simulink model "LGS_allFaultsDeselected"  (R2019b)
settings: Solver=FixedStepDiscrete  StartTime=0.0  StopTime=45.0  FixedStep=0.1  RelTol=1e-3
model workspace (MAT data in the model file):
  fipData : object (value not decoded)
  fipName : object (value not decoded)
  stepSize = 0.1
libraries: LibFaultInjectionControls x190, commrandsrc3 x70, simulink x3, LibFailureCondition x1
(part 4 of 41)

== system LGS_allFaultsDeselected/sensor up down handle/FIP2 ==
  In1 : Inport
  Handle sensor FIP2 : Subsystem  mask(FailureInjectionPoint){}
      mask help: FailureInjectionPoint
      mask init: same as LGS_allFaultsDeselected/Analogical switch and general electro-valve and pressure sensor/Analogical switch/Analog Switch FIP
      settings: OpenFcn=|
      | open_system(gcb,'mask');
      | 
      | treeValues = FailureInjectionPointHelper.getAllFmAndParamsAsTreeString(gcb);
      | mo = Simulink.Mask.get(gcb);
      | dc = mo.getDialogControl('GbFmInfo');
      | treeView = dc.getDialogControl('TreeViewFM');
      | treeView.TreeItems = {};
      | treeView.TreeItems = treeValues;
      mask Help: FailureInjectionPoint
      mask DialogControl Control7 Prompt: Containing Failure Modes
      mask DialogControl BtnMoveUp Prompt: Move up
      mask DialogControl BtnMoveUp Callback:
      | %Get name of the failure mode block
      | mo = Simulink.Mask.get(gcb);
      | dc = mo.getDialogControl('GbFmInfo');
      | treeView = dc.getDialogControl('TreeViewFM');
      | try
      |     a = treeView.getSelectedItems();
      |     p = split(a, '/'); %name of failure mode block is p{1}
      | catch
      |     return;
      | end
      | 
      | %Save port handles
      | lh = get_param([gcb,'/',p{1}],'LineHandles');
      | ph = get_param([gcb,'/',p{1}],'PortHandles');
      | this_in = ph.Inport(1);
      | this_out = ph.Outport(1);
      | 
      | last_block = get_param(lh.Inport(1),'SrcBlockHandle');
      | last_block_type = get_param(last_block,'BlockType');
      | if strcmp(last_block_type,'Inport')
      |     return;
      | end
      | lb_lh = get_param(last_block,'LineHandles');
      | 
      | last_out = get_param(lh.Inport(1),'SrcPortHandle');
      | last_in = get_param(lb_lh.Inport(1),'DstPortHandle');
      | next_to_last_out = get_param(lb_lh.Inport(1),'SrcPortHandle');
      | next_in = get_param(lh.Outport(1),'DstPortHandle');
      | 
      | %Delete connecting lines
      | delete_line(lh.Inport(1));
      | delete_line(lh.Outport(1));
      | delete_line(lb_lh.Inport(1));
      | 
      | % Generate new lines
      | add_line(gcb, last_out, next_in, 'autorouting', 'smart');
      | add_line(gcb, this_out, last_in, 'autorouting', 'smart');
      | add_line(gcb, next_to_last_out, this_in, 'autorouting', 'smart');
      | 
      | %Rearrange system
      | Simulink.BlockDiagram.arrangeSystem(gcb);
      | 
      | %Refresh
      | treeValues = FailureInjectionPointHelper.getAllFmAndParamsAsTreeString(gcb);
      | mo = Simulink.Mask.get(gcb);
      | dc = mo.getDialogControl('GbFmInfo');
      | treeView = dc.getDialogControl('TreeViewFM');
      | treeView.TreeItems = {};
      | treeView.TreeItems = treeValues;
      mask DialogControl BtnMoveDown Prompt: Move down
      mask DialogControl BtnMoveDown Callback:
      | %Get name of the failure mode block
      | mo = Simulink.Mask.get(gcb);
      | dc = mo.getDialogControl('GbFmInfo');
      | treeView = dc.getDialogControl('TreeViewFM');
      | try
      |     a = treeView.getSelectedItems();
      |     p = split(a, '/'); %name of failure mode block is p{1}
      | catch
      |     return;
      | end
      | 
      | %Save port handles
      | lh = get_param([gcb,'/',p{1}],'LineHandles');
      | ph = get_param([gcb,'/',p{1}],'PortHandles');
      | this_in = ph.Inport(1);
      | this_out = ph.Outport(1);
      | 
      | next_block = get_param(lh.Outport(1),'DstBlockHandle');
      | next_block_type = get_param(next_block,'BlockType');
      | if strcmp(next_block_type,'Outport')
      |     return;
      | end
      | nb_lh = get_param(next_block,'LineHandles');
      | 
      | last_out = get_param(lh.Inport(1),'SrcPortHandle');
      | next_out = get_param(nb_lh.Outport(1),'SrcPortHandle');
      | next_but_one_in = get_param(nb_lh.Outport(1),'DstPortHandle');
      | next_in = get_param(lh.Outport(1),'DstPortHandle');
      | 
      | %Delete connecting lines
      | delete_line(lh.Inport(1));
      | delete_line(lh.Outport(1));
      | delete_line(nb_lh.Outport(1));
      | 
      | % Generate new lines
      | add_line(gcb, last_out, next_in, 'autorouting', 'smart');
      | add_line(gcb, next_out, this_in, 'autorouting', 'smart');
      | add_line(gcb, this_out, next_but_one_in, 'autorouting', 'smart');
      | 
      | %Rearrange system
      | Simulink.BlockDiagram.arrangeSystem(gcb);
      | 
      | %Refresh
      | treeValues = FailureInjectionPointHelper.getAllFmAndParamsAsTreeString(gcb);
      | mo = Simulink.Mask.get(gcb);
      | dc = mo.getDialogControl('GbFmInfo');
      | treeView = dc.getDialogControl('TreeViewFM');
      | treeView.TreeItems = {};
      | treeView.TreeItems = treeValues;
      mask DialogControl TreeViewFM Prompt: Failure Mode Information
      mask DialogControl BtnOpen Prompt: Open FIP
      mask DialogControl BtnOpen Callback: open_system(gcb,'force');
      mask DialogControl BtnNew Prompt: New
      mask DialogControl BtnNew Callback:
      | dialog_fipManager_single(gcb, '');
      | 
      | %Enable move, edit, delete buttons
      | mo = Simulink.Mask.get(gcb);
      | mo.getDialogControl('BtnMoveUp').Enabled = 'on';
      | mo.getDialogControl('BtnMoveDown').Enabled = 'on';
      | mo.getDialogControl('BtnEdit').Enabled = 'on';
      | mo.getDialogControl('BtnDelete').Enabled = 'on';
      mask DialogControl BtnEdit Prompt: Edit
      mask DialogControl BtnEdit Callback:
      | mo = Simulink.Mask.get(gcb);
      | dc = mo.getDialogControl('GbFmInfo');
      | treeView = dc.getDialogControl('TreeViewFM');
      | try
      |     a = treeView.getSelectedItems();
      |     p = split(a, '/');
      | catch
      |     return;
      | end
      | dialog_fipManager_single(gcb, p{1});
      mask DialogControl BtnDelete Prompt: Delete
      mask DialogControl BtnDelete Callback:
      | %Get name of the failure mode block
      | mo = Simulink.Mask.get(gcb);
      | dc = mo.getDialogControl('GbFmInfo');
      | treeView = dc.getDialogControl('TreeViewFM');
      | try
      |     a = treeView.getSelectedItems();
      |     p = split(a, '/'); %name of failure mode block is p{1}
      | catch
      |     return;
      | end
      | 
      | %Save outport handle of the last and inport handle of the next block
      | lh = get_param([gcb,'/',p{1}],'LineHandles');
      | last_out = get_param(lh.Inport(1),'SrcPortHandle');
      | next_in = get_param(lh.Outport(1),'DstPortHandle');
      | 
      | %Delete connecting lines and failure mode block
      | delete_line(lh.Inport(1));
      | delete_line(lh.Outport(1));
      | fm_handle = get_param([gcb,'/',p{1}],'Handle');
      | delete_block(fm_handle);
      | 
      | % Generate new line from outport last to inport next
      | add_line(gcb, last_out, next_in, 'autorouting', 'smart');
      | 
      | %Rearrange system
      | Simulink.BlockDiagram.arrangeSystem(gcb);
      | 
      | %Disable move, edit, delete buttons in case all FMs are deleted
      | last_block = get_param(last_out,'Parent');
      | last_is_inport = strcmp(get_param(last_block,'BlockType'),'Inport');
      | next_block = get_param(next_in,'Parent');
      | next_is_outport = strcmp(get_param(next_block,'BlockType'),'Outport');
      | if (last_is_inport && next_is_outport)
      |     mo.getDialogControl('BtnMoveUp').Enabled = 'off';
      |     mo.getDialogControl('BtnMoveDown').Enabled = 'off';
      |     mo.getDialogControl('BtnEdit').Enabled = 'off';
      |     mo.getDialogControl('BtnDelete').Enabled = 'off';
      | end
      | 
      | %Refresh
      | treeValues = FailureInjectionPointHelper.getAllFmAndParamsAsTreeString(gcb);
      | mo = Simulink.Mask.get(gcb);
      | dc = mo.getDialogControl('GbFmInfo');
      | treeView = dc.getDialogControl('TreeViewFM');
      | treeView.TreeItems = {};
      | treeView.TreeItems = treeValues;
      mask DialogControl BtnRefresh Prompt: Refresh
      mask DialogControl BtnRefresh Callback:
      | set_param(gcb,'LinkStatus','none');
      | 
      | treeValues = FailureInjectionPointHelper.getAllFmAndParamsAsTreeString(gcb);
      | mo = Simulink.Mask.get(gcb);
      | dc = mo.getDialogControl('GbFmInfo');
      | treeView = dc.getDialogControl('TreeViewFM');
      | treeView.TreeItems = {};
      | treeView.TreeItems = treeValues;
      mask Display: image('icons/failure_injection_point.png','center')
  Out1 : Outport
  wires:
  In1/1 -> Handle sensor FIP2/1(In1)
  Handle sensor FIP2/1(Out1) -> Out1/1

== system LGS_allFaultsDeselected/sensor up down handle/FIP3 ==
  In1 : Inport
  Handle sensor FIP3 : Subsystem  mask(FailureInjectionPoint){}
      mask help: FailureInjectionPoint
      mask init: same as LGS_allFaultsDeselected/Analogical switch and general electro-valve and pressure sensor/Analogical switch/Analog Switch FIP
      settings: OpenFcn=|
      | open_system(gcb,'mask');
      | 
      | treeValues = FailureInjectionPointHelper.getAllFmAndParamsAsTreeString(gcb);
      | mo = Simulink.Mask.get(gcb);
      | dc = mo.getDialogControl('GbFmInfo');
      | treeView = dc.getDialogControl('TreeViewFM');
      | treeView.TreeItems = {};
      | treeView.TreeItems = treeValues;
      mask Help: FailureInjectionPoint
      mask DialogControl Control7 Prompt: Containing Failure Modes
      mask DialogControl BtnMoveUp Prompt: Move up
      mask DialogControl BtnMoveUp Callback:
      | %Get name of the failure mode block
      | mo = Simulink.Mask.get(gcb);
      | dc = mo.getDialogControl('GbFmInfo');
      | treeView = dc.getDialogControl('TreeViewFM');
      | try
      |     a = treeView.getSelectedItems();
      |     p = split(a, '/'); %name of failure mode block is p{1}
      | catch
      |     return;
      | end
      | 
      | %Save port handles
      | lh = get_param([gcb,'/',p{1}],'LineHandles');
      | ph = get_param([gcb,'/',p{1}],'PortHandles');
      | this_in = ph.Inport(1);
      | this_out = ph.Outport(1);
      | 
      | last_block = get_param(lh.Inport(1),'SrcBlockHandle');
      | last_block_type = get_param(last_block,'BlockType');
      | if strcmp(last_block_type,'Inport')
      |     return;
      | end
      | lb_lh = get_param(last_block,'LineHandles');
      | 
      | last_out = get_param(lh.Inport(1),'SrcPortHandle');
      | last_in = get_param(lb_lh.Inport(1),'DstPortHandle');
      | next_to_last_out = get_param(lb_lh.Inport(1),'SrcPortHandle');
      | next_in = get_param(lh.Outport(1),'DstPortHandle');
      | 
      | %Delete connecting lines
      | delete_line(lh.Inport(1));
      | delete_line(lh.Outport(1));
      | delete_line(lb_lh.Inport(1));
      | 
      | % Generate new lines
      | add_line(gcb, last_out, next_in, 'autorouting', 'smart');
      | add_line(gcb, this_out, last_in, 'autorouting', 'smart');
      | add_line(gcb, next_to_last_out, this_in, 'autorouting', 'smart');
      | 
      | %Rearrange system
      | Simulink.BlockDiagram.arrangeSystem(gcb);
      | 
      | %Refresh
      | treeValues = FailureInjectionPointHelper.getAllFmAndParamsAsTreeString(gcb);
      | mo = Simulink.Mask.get(gcb);
      | dc = mo.getDialogControl('GbFmInfo');
      | treeView = dc.getDialogControl('TreeViewFM');
      | treeView.TreeItems = {};
      | treeView.TreeItems = treeValues;
      mask DialogControl BtnMoveDown Prompt: Move down
      mask DialogControl BtnMoveDown Callback:
      | %Get name of the failure mode block
      | mo = Simulink.Mask.get(gcb);
      | dc = mo.getDialogControl('GbFmInfo');
      | treeView = dc.getDialogControl('TreeViewFM');
      | try
      |     a = treeView.getSelectedItems();
      |     p = split(a, '/'); %name of failure mode block is p{1}
      | catch
      |     return;
      | end
      | 
      | %Save port handles
      | lh = get_param([gcb,'/',p{1}],'LineHandles');
      | ph = get_param([gcb,'/',p{1}],'PortHandles');
      | this_in = ph.Inport(1);
      | this_out = ph.Outport(1);
      | 
      | next_block = get_param(lh.Outport(1),'DstBlockHandle');
      | next_block_type = get_param(next_block,'BlockType');
      | if strcmp(next_block_type,'Outport')
      |     return;
      | end
      | nb_lh = get_param(next_block,'LineHandles');
      | 
      | last_out = get_param(lh.Inport(1),'SrcPortHandle');
      | next_out = get_param(nb_lh.Outport(1),'SrcPortHandle');
      | next_but_one_in = get_param(nb_lh.Outport(1),'DstPortHandle');
      | next_in = get_param(lh.Outport(1),'DstPortHandle');
      | 
      | %Delete connecting lines
      | delete_line(lh.Inport(1));
      | delete_line(lh.Outport(1));
      | delete_line(nb_lh.Outport(1));
      | 
      | % Generate new lines
      | add_line(gcb, last_out, next_in, 'autorouting', 'smart');
      | add_line(gcb, next_out, this_in, 'autorouting', 'smart');
      | add_line(gcb, this_out, next_but_one_in, 'autorouting', 'smart');
      | 
      | %Rearrange system
      | Simulink.BlockDiagram.arrangeSystem(gcb);
      | 
      | %Refresh
      | treeValues = FailureInjectionPointHelper.getAllFmAndParamsAsTreeString(gcb);
      | mo = Simulink.Mask.get(gcb);
      | dc = mo.getDialogControl('GbFmInfo');
      | treeView = dc.getDialogControl('TreeViewFM');
      | treeView.TreeItems = {};
      | treeView.TreeItems = treeValues;
      mask DialogControl TreeViewFM Prompt: Failure Mode Information
      mask DialogControl BtnOpen Prompt: Open FIP
      mask DialogControl BtnOpen Callback: open_system(gcb,'force');
      mask DialogControl BtnNew Prompt: New
      mask DialogControl BtnNew Callback:
      | dialog_fipManager_single(gcb, '');
      | 
      | %Enable move, edit, delete buttons
      | mo = Simulink.Mask.get(gcb);
      | mo.getDialogControl('BtnMoveUp').Enabled = 'on';
      | mo.getDialogControl('BtnMoveDown').Enabled = 'on';
      | mo.getDialogControl('BtnEdit').Enabled = 'on';
      | mo.getDialogControl('BtnDelete').Enabled = 'on';
      mask DialogControl BtnEdit Prompt: Edit
      mask DialogControl BtnEdit Callback:
      | mo = Simulink.Mask.get(gcb);
      | dc = mo.getDialogControl('GbFmInfo');
      | treeView = dc.getDialogControl('TreeViewFM');
      | try
      |     a = treeView.getSelectedItems();
      |     p = split(a, '/');
      | catch
      |     return;
      | end
      | dialog_fipManager_single(gcb, p{1});
      mask DialogControl BtnDelete Prompt: Delete
      mask DialogControl BtnDelete Callback:
      | %Get name of the failure mode block
      | mo = Simulink.Mask.get(gcb);
      | dc = mo.getDialogControl('GbFmInfo');
      | treeView = dc.getDialogControl('TreeViewFM');
      | try
      |     a = treeView.getSelectedItems();
      |     p = split(a, '/'); %name of failure mode block is p{1}
      | catch
      |     return;
      | end
      | 
      | %Save outport handle of the last and inport handle of the next block
      | lh = get_param([gcb,'/',p{1}],'LineHandles');
      | last_out = get_param(lh.Inport(1),'SrcPortHandle');
      | next_in = get_param(lh.Outport(1),'DstPortHandle');
      | 
      | %Delete connecting lines and failure mode block
      | delete_line(lh.Inport(1));
      | delete_line(lh.Outport(1));
      | fm_handle = get_param([gcb,'/',p{1}],'Handle');
      | delete_block(fm_handle);
      | 
      | % Generate new line from outport last to inport next
      | add_line(gcb, last_out, next_in, 'autorouting', 'smart');
      | 
      | %Rearrange system
      | Simulink.BlockDiagram.arrangeSystem(gcb);
      | 
      | %Disable move, edit, delete buttons in case all FMs are deleted
      | last_block = get_param(last_out,'Parent');
      | last_is_inport = strcmp(get_param(last_block,'BlockType'),'Inport');
      | next_block = get_param(next_in,'Parent');
      | next_is_outport = strcmp(get_param(next_block,'BlockType'),'Outport');
      | if (last_is_inport && next_is_outport)
      |     mo.getDialogControl('BtnMoveUp').Enabled = 'off';
      |     mo.getDialogControl('BtnMoveDown').Enabled = 'off';
      |     mo.getDialogControl('BtnEdit').Enabled = 'off';
      |     mo.getDialogControl('BtnDelete').Enabled = 'off';
      | end
      | 
      | %Refresh
      | treeValues = FailureInjectionPointHelper.getAllFmAndParamsAsTreeString(gcb);
      | mo = Simulink.Mask.get(gcb);
      | dc = mo.getDialogControl('GbFmInfo');
      | treeView = dc.getDialogControl('TreeViewFM');
      | treeView.TreeItems = {};
      | treeView.TreeItems = treeValues;
      mask DialogControl BtnRefresh Prompt: Refresh
      mask DialogControl BtnRefresh Callback:
      | set_param(gcb,'LinkStatus','none');
      | 
      | treeValues = FailureInjectionPointHelper.getAllFmAndParamsAsTreeString(gcb);
      | mo = Simulink.Mask.get(gcb);
      | dc = mo.getDialogControl('GbFmInfo');
      | treeView = dc.getDialogControl('TreeViewFM');
      | treeView.TreeItems = {};
      | treeView.TreeItems = treeValues;
      mask Display: image('icons/failure_injection_point.png','center')
  Out1 : Outport
  wires:
  In1/1 -> Handle sensor FIP3/1(In1)
  Handle sensor FIP3/1(Out1) -> Out1/1

== system LGS_allFaultsDeselected/Analogical switch and general electro-valve and pressure sensor/Analogical switch/Analog Switch FIP ==
  In1 : Inport
  Blocked closed : Subsystem  mask(FailureMode){isActive=off, isDSF=off, Value=true, FailureRate=1.0E-3, useDefaultMt_copy=off, MaintenanceTask=0, useDefaultMt=off, RiskTime=0, useDefaultRt=off, File=[], DSFjson=JSON}
      mask prompts: isActive "is Active"; isDSF "DSF Trigger"; Value "Bool Value"; useDefaultMt_copy "set"; useDefaultMt "set"; useDefaultRt "set"
      mask TypeOptions isActive: Trigger FIP/Active
      mask TypeOptions isDSF: Trigger FIP/isDSF
      mask Callback isDSF:
      | a = Simulink.Mask.get(gcb);
      | disp(a);
      | d = a.DialogControls();
      | disp(d);
      | for i = 1:size(d,2)
      |     if strcmp(d(i).Name, 'ParameterGroupVar')
      |         basicFip_ctrl = d(i).getDialogControl('BasicFipParam');
      |         dsFip_ctrl = d(i).getDialogControl('DSFipParam');
      | 
      |         if strcmp(get_param(gcb, 'isDSF'), 'on')
      | %            basicFip_ctrl.Visible = 'off';
      |             basicFip_ctrl.Enabled = 'off';
      | 
      |             dsFip_ctrl.Enabled = 'on';
      | %            dsFip_ctrl.Visible = 'on';
      |         else
      |             basicFip_ctrl.Enabled = 'on';
      | %            basicFip_ctrl.Visible = 'on';
      | 
      | %            dsFip_ctrl.Visible = 'off';
      |             dsFip_ctrl.Enabled = 'off';
      |         end
      |     end
      | end
      mask TypeOptions Value: CommitValue/Value
      mask TypeOptions FailureRate: Trigger FIP/FailureRate
      mask Callback useDefaultMt_copy:
      | a = Simulink.Mask.get(gcb);
      | d = a.Parameters();
      | for i = 1:size(d,2)
      |     if strcmp(d(i).Name, 'MaintenanceTask')
      |         if strcmp(get_param(gcb, 'useDefaultMt'), 'off')
      |             set_param(gcb,'MaintenanceTask', '0')
      |             d(i).Enabled = 'off';
      |         else
      |             d(i).Enabled = 'on';
      |         end
      |     end
      | end
      mask TypeOptions MaintenanceTask: Trigger FIP/MaintenanceTask
      mask Callback useDefaultMt:
      | a = Simulink.Mask.get(gcb);
      | d = a.Parameters();
      | for i = 1:size(d,2)
      |     if strcmp(d(i).Name, 'MaintenanceTask')
      |         if strcmp(get_param(gcb, 'useDefaultMt'), 'off')
      |             set_param(gcb,'MaintenanceTask', '0')
      |             d(i).Enabled = 'off';
      |         else
      |             d(i).Enabled = 'on';
      |         end
      |     end
      | end
      mask TypeOptions RiskTime: Trigger FIP/RiskTime
      mask Callback useDefaultRt:
      | a = Simulink.Mask.get(gcb);
      | d = a.Parameters();
      | for i = 1:size(d,2)
      |     if strcmp(d(i).Name, 'RiskTime')
      |         if strcmp(get_param(gcb, 'useDefaultRt'), 'off')
      |             set_param(gcb,'RiskTime', '0')
      |             d(i).Enabled = 'off';
      |         else
      |             d(i).Enabled = 'on';
      |         end
      |     end
      | end
      mask TypeOptions DSFjson: Trigger FIP/DSFjson
      mask DialogControl DescGroupVar Prompt: Bool
      mask DialogControl DescTextVar Prompt: Controls for a fault with boolean as result type
      mask DialogControl BasicFipBehavior Prompt: Failure Mode Behavior
      mask DialogControl BasicFipParamTab Prompt: Failure Mode Occurrence
      mask DialogControl BasicFipParam Prompt: Parameters
      mask DialogControl FailureRate_label Prompt: Failure Rate [1/h]
      mask DialogControl MaintenanceTask_label Prompt: Maintenance Task [h]
      mask DialogControl RiskTime_label Prompt: Risk time [h]
      mask DialogControl DSFipParamTab Prompt: Dependent System Information
      mask DialogControl DSFipParam Prompt: Parameters
      mask DialogControl LoadCSV Prompt: Browse
      mask DialogControl LoadCSV Callback:
      | [file,path,indx] = uigetfile('*.csv');
      | try
      |     set_param(gcb, 'File', append(path,file));
      |     file = fopen(append(path,file));
      | 
      |     fips = {};
      |     cutsets = {};
      | 
      |     line = fgetl(file);
      |     while ischar(line)
      |         disp(join([' > Processing: ',line]));
      |         splitString = split(line, ';');
      |         if isequal(splitString{1}, 'Cut set')
      |             disp('   > Found Cut set');
      |             cs = splitString(2:end-1);
      |             disp(cs);
      |             cutsets{end+1} = cs';
      |         else
      |             disp('   > Found FIP');
      |             if ~isequal("h", splitString(7))
      |                 disp('no time format except hour is supported');
      |             end
      |             fip = {};
      |             fip.id = splitString(1);
      |             fip.path = splitString(3);
      |             fip.rate = splitString(4);
      |             fip.checkInterval = splitString(6);
      |             disp(fip);
      |             fips{end+1} = fip;
      |         end
      |         line = fgetl(file);
      |     end
      | 
      |     fclose(file);
      | 
      |     DSF = {};
      |     DSF.fips = fips;
      |     DSF.cutsets = cutsets;
      | 
      |     VarCSText = jsonencode(DSF);
      |     set_param(gcb, 'DSFjson', VarCSText);
      | catch
      | end
  Blocked open : Subsystem  mask(FailureMode){isActive=off, isDSF=off, Value=false, FailureRate=1.0E-3, useDefaultMt_copy=off, MaintenanceTask=0, useDefaultMt=off, RiskTime=0, useDefaultRt=off, File=[], DSFjson=JSON}
      mask prompts: isActive "is Active"; isDSF "DSF Trigger"; Value "Bool Value"; useDefaultMt_copy "set"; useDefaultMt "set"; useDefaultRt "set"
      mask TypeOptions isActive: Trigger FIP/Active
      mask TypeOptions isDSF: Trigger FIP/isDSF
      mask Callback isDSF:
      | a = Simulink.Mask.get(gcb);
      | disp(a);
      | d = a.DialogControls();
      | disp(d);
      | for i = 1:size(d,2)
      |     if strcmp(d(i).Name, 'ParameterGroupVar')
      |         basicFip_ctrl = d(i).getDialogControl('BasicFipParam');
      |         dsFip_ctrl = d(i).getDialogControl('DSFipParam');
      | 
      |         if strcmp(get_param(gcb, 'isDSF'), 'on')
      | %            basicFip_ctrl.Visible = 'off';
      |             basicFip_ctrl.Enabled = 'off';
      | 
      |             dsFip_ctrl.Enabled = 'on';
      | %            dsFip_ctrl.Visible = 'on';
      |         else
      |             basicFip_ctrl.Enabled = 'on';
      | %            basicFip_ctrl.Visible = 'on';
      | 
      | %            dsFip_ctrl.Visible = 'off';
      |             dsFip_ctrl.Enabled = 'off';
      |         end
      |     end
      | end
      mask TypeOptions Value: CommitValue/Value
      mask TypeOptions FailureRate: Trigger FIP/FailureRate
      mask Callback useDefaultMt_copy:
      | a = Simulink.Mask.get(gcb);
      | d = a.Parameters();
      | for i = 1:size(d,2)
      |     if strcmp(d(i).Name, 'MaintenanceTask')
      |         if strcmp(get_param(gcb, 'useDefaultMt'), 'off')
      |             set_param(gcb,'MaintenanceTask', '0')
      |             d(i).Enabled = 'off';
      |         else
      |             d(i).Enabled = 'on';
      |         end
      |     end
      | end
      mask TypeOptions MaintenanceTask: Trigger FIP/MaintenanceTask
      mask Callback useDefaultMt:
      | a = Simulink.Mask.get(gcb);
      | d = a.Parameters();
      | for i = 1:size(d,2)
      |     if strcmp(d(i).Name, 'MaintenanceTask')
      |         if strcmp(get_param(gcb, 'useDefaultMt'), 'off')
      |             set_param(gcb,'MaintenanceTask', '0')
      |             d(i).Enabled = 'off';
      |         else
      |             d(i).Enabled = 'on';
      |         end
      |     end
      | end
      mask TypeOptions RiskTime: Trigger FIP/RiskTime
      mask Callback useDefaultRt:
      | a = Simulink.Mask.get(gcb);
      | d = a.Parameters();
      | for i = 1:size(d,2)
      |     if strcmp(d(i).Name, 'RiskTime')
      |         if strcmp(get_param(gcb, 'useDefaultRt'), 'off')
      |             set_param(gcb,'RiskTime', '0')
      |             d(i).Enabled = 'off';
      |         else
      |             d(i).Enabled = 'on';
      |         end
      |     end
      | end
      mask TypeOptions DSFjson: Trigger FIP/DSFjson
      mask DialogControl DescGroupVar Prompt: Bool
      mask DialogControl DescTextVar Prompt: Controls for a fault with boolean as result type
      mask DialogControl BasicFipBehavior Prompt: Failure Mode Behavior
      mask DialogControl BasicFipParamTab Prompt: Failure Mode Occurrence
      mask DialogControl BasicFipParam Prompt: Parameters
      mask DialogControl FailureRate_label Prompt: Failure Rate [1/h]
      mask DialogControl MaintenanceTask_label Prompt: Maintenance Task [h]
      mask DialogControl RiskTime_label Prompt: Risk time [h]
      mask DialogControl DSFipParamTab Prompt: Dependent System Information
      mask DialogControl DSFipParam Prompt: Parameters
      mask DialogControl LoadCSV Prompt: Browse
      mask DialogControl LoadCSV Callback:
      | [file,path,indx] = uigetfile('*.csv');
      | try
      |     set_param(gcb, 'File', append(path,file));
      |     file = fopen(append(path,file));
      | 
      |     fips = {};
      |     cutsets = {};
      | 
      |     line = fgetl(file);
      |     while ischar(line)
      |         disp(join([' > Processing: ',line]));
      |         splitString = split(line, ';');
      |         if isequal(splitString{1}, 'Cut set')
      |             disp('   > Found Cut set');
      |             cs = splitString(2:end-1);
      |             disp(cs);
      |             cutsets{end+1} = cs';
      |         else
      |             disp('   > Found FIP');
      |             if ~isequal("h", splitString(7))
      |                 disp('no time format except hour is supported');
      |             end
      |             fip = {};
      |             fip.id = splitString(1);
      |             fip.path = splitString(3);
      |             fip.rate = splitString(4);
      |             fip.checkInterval = splitString(6);
      |             disp(fip);
      |             fips{end+1} = fip;
      |         end
      |         line = fgetl(file);
      |     end
      | 
      |     fclose(file);
      | 
      |     DSF = {};
      |     DSF.fips = fips;
      |     DSF.cutsets = cutsets;
      | 
      |     VarCSText = jsonencode(DSF);
      |     set_param(gcb, 'DSFjson', VarCSText);
      | catch
      | end
  Out1 : Outport
  wires:
  Blocked closed/1(Out1) -> Blocked open/1(In1)
  In1/1 -> Blocked closed/1(In1)
  Blocked open/1(Out1) -> Out1/1

== system LGS_allFaultsDeselected/Analogical switch and general electro-valve and pressure sensor/General EV/General EV FIP ==
  In1 : Inport
  Blocked closed : Subsystem  mask(FailureMode){isActive=off, isDSF=off, Value=false, FailureRate=1.0E-3, useDefaultMt_copy=off, MaintenanceTask=0, useDefaultMt=off, RiskTime=0, useDefaultRt=off, File=[], DSFjson=JSON}
      mask prompts: isActive "is Active"; isDSF "DSF Trigger"; Value "Bool Value"; useDefaultMt_copy "set"; useDefaultMt "set"; useDefaultRt "set"
      mask TypeOptions isActive: Trigger FIP/Active
      mask TypeOptions isDSF: Trigger FIP/isDSF
      mask Callback isDSF:
      | a = Simulink.Mask.get(gcb);
      | disp(a);
      | d = a.DialogControls();
      | disp(d);
      | for i = 1:size(d,2)
      |     if strcmp(d(i).Name, 'ParameterGroupVar')
      |         basicFip_ctrl = d(i).getDialogControl('BasicFipParam');
      |         dsFip_ctrl = d(i).getDialogControl('DSFipParam');
      | 
      |         if strcmp(get_param(gcb, 'isDSF'), 'on')
      | %            basicFip_ctrl.Visible = 'off';
      |             basicFip_ctrl.Enabled = 'off';
      | 
      |             dsFip_ctrl.Enabled = 'on';
      | %            dsFip_ctrl.Visible = 'on';
      |         else
      |             basicFip_ctrl.Enabled = 'on';
      | %            basicFip_ctrl.Visible = 'on';
      | 
      | %            dsFip_ctrl.Visible = 'off';
      |             dsFip_ctrl.Enabled = 'off';
      |         end
      |     end
      | end
      mask TypeOptions Value: CommitValue/Value
      mask TypeOptions FailureRate: Trigger FIP/FailureRate
      mask Callback useDefaultMt_copy:
      | a = Simulink.Mask.get(gcb);
      | d = a.Parameters();
      | for i = 1:size(d,2)
      |     if strcmp(d(i).Name, 'MaintenanceTask')
      |         if strcmp(get_param(gcb, 'useDefaultMt'), 'off')
      |             set_param(gcb,'MaintenanceTask', '0')
      |             d(i).Enabled = 'off';
      |         else
      |             d(i).Enabled = 'on';
      |         end
      |     end
      | end
      mask TypeOptions MaintenanceTask: Trigger FIP/MaintenanceTask
      mask Callback useDefaultMt:
      | a = Simulink.Mask.get(gcb);
      | d = a.Parameters();
      | for i = 1:size(d,2)
      |     if strcmp(d(i).Name, 'MaintenanceTask')
      |         if strcmp(get_param(gcb, 'useDefaultMt'), 'off')
      |             set_param(gcb,'MaintenanceTask', '0')
      |             d(i).Enabled = 'off';
      |         else
      |             d(i).Enabled = 'on';
      |         end
      |     end
      | end
      mask TypeOptions RiskTime: Trigger FIP/RiskTime
      mask Callback useDefaultRt:
      | a = Simulink.Mask.get(gcb);
      | d = a.Parameters();
      | for i = 1:size(d,2)
      |     if strcmp(d(i).Name, 'RiskTime')
      |         if strcmp(get_param(gcb, 'useDefaultRt'), 'off')
      |             set_param(gcb,'RiskTime', '0')
      |             d(i).Enabled = 'off';
      |         else
      |             d(i).Enabled = 'on';
      |         end
      |     end
      | end
      mask TypeOptions DSFjson: Trigger FIP/DSFjson
      mask DialogControl DescGroupVar Prompt: Bool
      mask DialogControl DescTextVar Prompt: Controls for a fault with boolean as result type
      mask DialogControl BasicFipBehavior Prompt: Failure Mode Behavior
      mask DialogControl BasicFipParamTab Prompt: Failure Mode Occurrence
      mask DialogControl BasicFipParam Prompt: Parameters
      mask DialogControl FailureRate_label Prompt: Failure Rate [1/h]
      mask DialogControl MaintenanceTask_label Prompt: Maintenance Task [h]
      mask DialogControl RiskTime_label Prompt: Risk time [h]
      mask DialogControl DSFipParamTab Prompt: Dependent System Information
      mask DialogControl DSFipParam Prompt: Parameters
      mask DialogControl LoadCSV Prompt: Browse
      mask DialogControl LoadCSV Callback:
      | [file,path,indx] = uigetfile('*.csv');
      | try
      |     set_param(gcb, 'File', append(path,file));
      |     file = fopen(append(path,file));
      | 
      |     fips = {};
      |     cutsets = {};
      | 
      |     line = fgetl(file);
      |     while ischar(line)
      |         disp(join([' > Processing: ',line]));
      |         splitString = split(line, ';');
      |         if isequal(splitString{1}, 'Cut set')
      |             disp('   > Found Cut set');
      |             cs = splitString(2:end-1);
      |             disp(cs);
      |             cutsets{end+1} = cs';
      |         else
      |             disp('   > Found FIP');
      |             if ~isequal("h", splitString(7))
      |                 disp('no time format except hour is supported');
      |             end
      |             fip = {};
      |             fip.id = splitString(1);
      |             fip.path = splitString(3);
      |             fip.rate = splitString(4);
      |             fip.checkInterval = splitString(6);
      |             disp(fip);
      |             fips{end+1} = fip;
      |         end
      |         line = fgetl(file);
      |     end
      | 
      |     fclose(file);
      | 
      |     DSF = {};
      |     DSF.fips = fips;
      |     DSF.cutsets = cutsets;
      | 
      |     VarCSText = jsonencode(DSF);
      |     set_param(gcb, 'DSFjson', VarCSText);
      | catch
      | end
  Blocked open : Subsystem  mask(FailureMode){isActive=off, isDSF=off, Value=true, FailureRate=1.0E-3, useDefaultMt_copy=off, MaintenanceTask=0, useDefaultMt=off, RiskTime=0, useDefaultRt=off, File=[], DSFjson=JSON}
      mask prompts: isActive "is Active"; isDSF "DSF Trigger"; Value "Bool Value"; useDefaultMt_copy "set"; useDefaultMt "set"; useDefaultRt "set"
      mask TypeOptions isActive: Trigger FIP/Active
      mask TypeOptions isDSF: Trigger FIP/isDSF
      mask Callback isDSF:
      | a = Simulink.Mask.get(gcb);
      | disp(a);
      | d = a.DialogControls();
      | disp(d);
      | for i = 1:size(d,2)
      |     if strcmp(d(i).Name, 'ParameterGroupVar')
      |         basicFip_ctrl = d(i).getDialogControl('BasicFipParam');
      |         dsFip_ctrl = d(i).getDialogControl('DSFipParam');
      | 
      |         if strcmp(get_param(gcb, 'isDSF'), 'on')
      | %            basicFip_ctrl.Visible = 'off';
      |             basicFip_ctrl.Enabled = 'off';
      | 
      |             dsFip_ctrl.Enabled = 'on';
      | %            dsFip_ctrl.Visible = 'on';
      |         else
      |             basicFip_ctrl.Enabled = 'on';
      | %            basicFip_ctrl.Visible = 'on';
      | 
      | %            dsFip_ctrl.Visible = 'off';
      |             dsFip_ctrl.Enabled = 'off';
      |         end
      |     end
      | end
      mask TypeOptions Value: CommitValue/Value
      mask TypeOptions FailureRate: Trigger FIP/FailureRate
      mask Callback useDefaultMt_copy:
      | a = Simulink.Mask.get(gcb);
      | d = a.Parameters();
      | for i = 1:size(d,2)
      |     if strcmp(d(i).Name, 'MaintenanceTask')
      |         if strcmp(get_param(gcb, 'useDefaultMt'), 'off')
      |             set_param(gcb,'MaintenanceTask', '0')
      |             d(i).Enabled = 'off';
      |         else
      |             d(i).Enabled = 'on';
      |         end
      |     end
      | end
      mask TypeOptions MaintenanceTask: Trigger FIP/MaintenanceTask
      mask Callback useDefaultMt:
      | a = Simulink.Mask.get(gcb);
      | d = a.Parameters();
      | for i = 1:size(d,2)
      |     if strcmp(d(i).Name, 'MaintenanceTask')
      |         if strcmp(get_param(gcb, 'useDefaultMt'), 'off')
      |             set_param(gcb,'MaintenanceTask', '0')
      |             d(i).Enabled = 'off';
      |         else
      |             d(i).Enabled = 'on';
      |         end
      |     end
      | end
      mask TypeOptions RiskTime: Trigger FIP/RiskTime
      mask Callback useDefaultRt:
      | a = Simulink.Mask.get(gcb);
      | d = a.Parameters();
      | for i = 1:size(d,2)
      |     if strcmp(d(i).Name, 'RiskTime')
      |         if strcmp(get_param(gcb, 'useDefaultRt'), 'off')
      |             set_param(gcb,'RiskTime', '0')
      |             d(i).Enabled = 'off';
      |         else
      |             d(i).Enabled = 'on';
      |         end
      |     end
      | end
      mask TypeOptions DSFjson: Trigger FIP/DSFjson
      mask DialogControl DescGroupVar Prompt: Bool
      mask DialogControl DescTextVar Prompt: Controls for a fault with boolean as result type
      mask DialogControl BasicFipBehavior Prompt: Failure Mode Behavior
      mask DialogControl BasicFipParamTab Prompt: Failure Mode Occurrence
      mask DialogControl BasicFipParam Prompt: Parameters
      mask DialogControl FailureRate_label Prompt: Failure Rate [1/h]
      mask DialogControl MaintenanceTask_label Prompt: Maintenance Task [h]
      mask DialogControl RiskTime_label Prompt: Risk time [h]
      mask DialogControl DSFipParamTab Prompt: Dependent System Information
      mask DialogControl DSFipParam Prompt: Parameters
      mask DialogControl LoadCSV Prompt: Browse
      mask DialogControl LoadCSV Callback:
      | [file,path,indx] = uigetfile('*.csv');
      | try
      |     set_param(gcb, 'File', append(path,file));
      |     file = fopen(append(path,file));
      | 
      |     fips = {};
      |     cutsets = {};
      | 
      |     line = fgetl(file);
      |     while ischar(line)
      |         disp(join([' > Processing: ',line]));
      |         splitString = split(line, ';');
      |         if isequal(splitString{1}, 'Cut set')
      |             disp('   > Found Cut set');
      |             cs = splitString(2:end-1);
      |             disp(cs);
      |             cutsets{end+1} = cs';
      |         else
      |             disp('   > Found FIP');
      |             if ~isequal("h", splitString(7))
      |                 disp('no time format except hour is supported');
      |             end
      |             fip = {};
      |             fip.id = splitString(1);
      |             fip.path = splitString(3);
      |             fip.rate = splitString(4);
      |             fip.checkInterval = splitString(6);
      |             disp(fip);
      |             fips{end+1} = fip;
      |         end
      |         line = fgetl(file);
      |     end
      | 
      |     fclose(file);
      | 
      |     DSF = {};
      |     DSF.fips = fips;
      |     DSF.cutsets = cutsets;
      | 
      |     VarCSText = jsonencode(DSF);
      |     set_param(gcb, 'DSFjson', VarCSText);
      | catch
      | end
  Out1 : Outport
  wires:
  Blocked open/1(Out1) -> Out1/1
  Blocked closed/1(Out1) -> Blocked open/1(In1)
  In1/1 -> Blocked closed/1(In1)

== system LGS_allFaultsDeselected/Analogical switch and general electro-valve and pressure sensor/sensor switch closed/FIP1 ==
  In1 : Inport
  Switch closed sensor FIP1 : Subsystem  mask(FailureInjectionPoint){}
      mask help: FailureInjectionPoint
      mask init: same as LGS_allFaultsDeselected/Analogical switch and general electro-valve and pressure sensor/Analogical switch/Analog Switch FIP
      settings: OpenFcn=|
      | open_system(gcb,'mask');
      | 
      | treeValues = FailureInjectionPointHelper.getAllFmAndParamsAsTreeString(gcb);
      | mo = Simulink.Mask.get(gcb);
      | dc = mo.getDialogControl('GbFmInfo');
      | treeView = dc.getDialogControl('TreeViewFM');
      | treeView.TreeItems = {};
      | treeView.TreeItems = treeValues;
      mask Help: FailureInjectionPoint
      mask DialogControl Control7 Prompt: Containing Failure Modes
      mask DialogControl BtnMoveUp Prompt: Move up
      mask DialogControl BtnMoveUp Callback:
      | %Get name of the failure mode block
      | mo = Simulink.Mask.get(gcb);
      | dc = mo.getDialogControl('GbFmInfo');
      | treeView = dc.getDialogControl('TreeViewFM');
      | try
      |     a = treeView.getSelectedItems();
      |     p = split(a, '/'); %name of failure mode block is p{1}
      | catch
      |     return;
      | end
      | 
      | %Save port handles
      | lh = get_param([gcb,'/',p{1}],'LineHandles');
      | ph = get_param([gcb,'/',p{1}],'PortHandles');
      | this_in = ph.Inport(1);
      | this_out = ph.Outport(1);
      | 
      | last_block = get_param(lh.Inport(1),'SrcBlockHandle');
      | last_block_type = get_param(last_block,'BlockType');
      | if strcmp(last_block_type,'Inport')
      |     return;
      | end
      | lb_lh = get_param(last_block,'LineHandles');
      | 
      | last_out = get_param(lh.Inport(1),'SrcPortHandle');
      | last_in = get_param(lb_lh.Inport(1),'DstPortHandle');
      | next_to_last_out = get_param(lb_lh.Inport(1),'SrcPortHandle');
      | next_in = get_param(lh.Outport(1),'DstPortHandle');
      | 
      | %Delete connecting lines
      | delete_line(lh.Inport(1));
      | delete_line(lh.Outport(1));
      | delete_line(lb_lh.Inport(1));
      | 
      | % Generate new lines
      | add_line(gcb, last_out, next_in, 'autorouting', 'smart');
      | add_line(gcb, this_out, last_in, 'autorouting', 'smart');
      | add_line(gcb, next_to_last_out, this_in, 'autorouting', 'smart');
      | 
      | %Rearrange system
      | Simulink.BlockDiagram.arrangeSystem(gcb);
      | 
      | %Refresh
      | treeValues = FailureInjectionPointHelper.getAllFmAndParamsAsTreeString(gcb);
      | mo = Simulink.Mask.get(gcb);
      | dc = mo.getDialogControl('GbFmInfo');
      | treeView = dc.getDialogControl('TreeViewFM');
      | treeView.TreeItems = {};
      | treeView.TreeItems = treeValues;
      mask DialogControl BtnMoveDown Prompt: Move down
      mask DialogControl BtnMoveDown Callback:
      | %Get name of the failure mode block
      | mo = Simulink.Mask.get(gcb);
      | dc = mo.getDialogControl('GbFmInfo');
      | treeView = dc.getDialogControl('TreeViewFM');
      | try
      |     a = treeView.getSelectedItems();
      |     p = split(a, '/'); %name of failure mode block is p{1}
      | catch
      |     return;
      | end
      | 
      | %Save port handles
      | lh = get_param([gcb,'/',p{1}],'LineHandles');
      | ph = get_param([gcb,'/',p{1}],'PortHandles');
      | this_in = ph.Inport(1);
      | this_out = ph.Outport(1);
      | 
      | next_block = get_param(lh.Outport(1),'DstBlockHandle');
      | next_block_type = get_param(next_block,'BlockType');
      | if strcmp(next_block_type,'Outport')
      |     return;
      | end
      | nb_lh = get_param(next_block,'LineHandles');
      | 
      | last_out = get_param(lh.Inport(1),'SrcPortHandle');
      | next_out = get_param(nb_lh.Outport(1),'SrcPortHandle');
      | next_but_one_in = get_param(nb_lh.Outport(1),'DstPortHandle');
      | next_in = get_param(lh.Outport(1),'DstPortHandle');
      | 
      | %Delete connecting lines
      | delete_line(lh.Inport(1));
      | delete_line(lh.Outport(1));
      | delete_line(nb_lh.Outport(1));
      | 
      | % Generate new lines
      | add_line(gcb, last_out, next_in, 'autorouting', 'smart');
      | add_line(gcb, next_out, this_in, 'autorouting', 'smart');
      | add_line(gcb, this_out, next_but_one_in, 'autorouting', 'smart');
      | 
      | %Rearrange system
      | Simulink.BlockDiagram.arrangeSystem(gcb);
      | 
      | %Refresh
      | treeValues = FailureInjectionPointHelper.getAllFmAndParamsAsTreeString(gcb);
      | mo = Simulink.Mask.get(gcb);
      | dc = mo.getDialogControl('GbFmInfo');
      | treeView = dc.getDialogControl('TreeViewFM');
      | treeView.TreeItems = {};
      | treeView.TreeItems = treeValues;
      mask DialogControl TreeViewFM Prompt: Failure Mode Information
      mask DialogControl BtnOpen Prompt: Open FIP
      mask DialogControl BtnOpen Callback: open_system(gcb,'force');
      mask DialogControl BtnNew Prompt: New
      mask DialogControl BtnNew Callback:
      | dialog_fipManager_single(gcb, '');
      | 
      | %Enable move, edit, delete buttons
      | mo = Simulink.Mask.get(gcb);
      | mo.getDialogControl('BtnMoveUp').Enabled = 'on';
      | mo.getDialogControl('BtnMoveDown').Enabled = 'on';
      | mo.getDialogControl('BtnEdit').Enabled = 'on';
      | mo.getDialogControl('BtnDelete').Enabled = 'on';
      mask DialogControl BtnEdit Prompt: Edit
      mask DialogControl BtnEdit Callback:
      | mo = Simulink.Mask.get(gcb);
      | dc = mo.getDialogControl('GbFmInfo');
      | treeView = dc.getDialogControl('TreeViewFM');
      | try
      |     a = treeView.getSelectedItems();
      |     p = split(a, '/');
      | catch
      |     return;
      | end
      | dialog_fipManager_single(gcb, p{1});
      mask DialogControl BtnDelete Prompt: Delete
      mask DialogControl BtnDelete Callback:
      | %Get name of the failure mode block
      | mo = Simulink.Mask.get(gcb);
      | dc = mo.getDialogControl('GbFmInfo');
      | treeView = dc.getDialogControl('TreeViewFM');
      | try
      |     a = treeView.getSelectedItems();
      |     p = split(a, '/'); %name of failure mode block is p{1}
      | catch
      |     return;
      | end
      | 
      | %Save outport handle of the last and inport handle of the next block
      | lh = get_param([gcb,'/',p{1}],'LineHandles');
      | last_out = get_param(lh.Inport(1),'SrcPortHandle');
      | next_in = get_param(lh.Outport(1),'DstPortHandle');
      | 
      | %Delete connecting lines and failure mode block
      | delete_line(lh.Inport(1));
      | delete_line(lh.Outport(1));
      | fm_handle = get_param([gcb,'/',p{1}],'Handle');
      | delete_block(fm_handle);
      | 
      | % Generate new line from outport last to inport next
      | add_line(gcb, last_out, next_in, 'autorouting', 'smart');
      | 
      | %Rearrange system
      | Simulink.BlockDiagram.arrangeSystem(gcb);
      | 
      | %Disable move, edit, delete buttons in case all FMs are deleted
      | last_block = get_param(last_out,'Parent');
      | last_is_inport = strcmp(get_param(last_block,'BlockType'),'Inport');
      | next_block = get_param(next_in,'Parent');
      | next_is_outport = strcmp(get_param(next_block,'BlockType'),'Outport');
      | if (last_is_inport && next_is_outport)
      |     mo.getDialogControl('BtnMoveUp').Enabled = 'off';
      |     mo.getDialogControl('BtnMoveDown').Enabled = 'off';
      |     mo.getDialogControl('BtnEdit').Enabled = 'off';
      |     mo.getDialogControl('BtnDelete').Enabled = 'off';
      | end
      | 
      | %Refresh
      | treeValues = FailureInjectionPointHelper.getAllFmAndParamsAsTreeString(gcb);
      | mo = Simulink.Mask.get(gcb);
      | dc = mo.getDialogControl('GbFmInfo');
      | treeView = dc.getDialogControl('TreeViewFM');
      | treeView.TreeItems = {};
      | treeView.TreeItems = treeValues;
      mask DialogControl BtnRefresh Prompt: Refresh
      mask DialogControl BtnRefresh Callback:
      | set_param(gcb,'LinkStatus','none');
      | 
      | treeValues = FailureInjectionPointHelper.getAllFmAndParamsAsTreeString(gcb);
      | mo = Simulink.Mask.get(gcb);
      | dc = mo.getDialogControl('GbFmInfo');
      | treeView = dc.getDialogControl('TreeViewFM');
      | treeView.TreeItems = {};
      | treeView.TreeItems = treeValues;
      mask Display: image('icons/failure_injection_point.png','center')
  Out1 : Outport
  wires:
  In1/1 -> Switch closed sensor FIP1/1(In1)
  Switch closed sensor FIP1/1(Out1) -> Out1/1
